simulink model "W2_prob2"  (R2020b)
settings: Solver=VariableStepAuto  StartTime=0.0  StopTime=10.0  RelTol=1e-3
values from neighbouring files (symbols this model uses):
  be = 2.0    [data2_dic.sldd]
  bv = 1.0    [data2_dic.sldd]
  Ie = 1.0    [data2_dic.sldd]
  Iv = 5.0    [data2_dic.sldd]
  R = 1.0    [data2_dic.sldd]
  Uk = 1.0    [data2_dic.sldd]
  Us = 1.5    [data2_dic.sldd]
settings Model: DataDictionary=data2_dic.sldd  Creator=deves  LastModifiedBy=deves
settings SolverCC: ZeroCrossAlgorithm=Adaptive
settings DebuggingCC: IgnoredZcDiagnostic=none

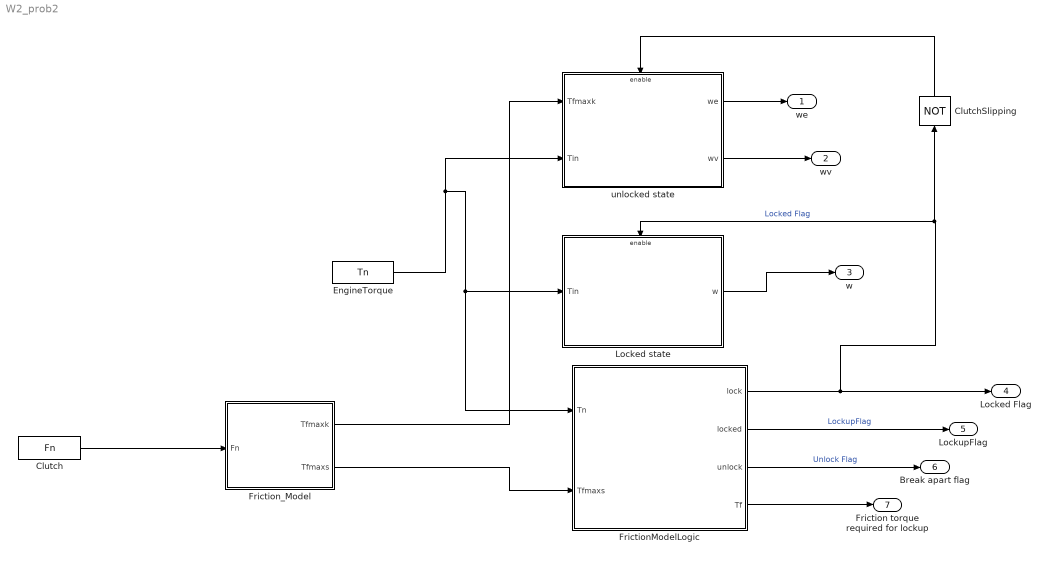
== system W2_prob2 ==
  Clutch : FromWorkspace  VariableName=Fn
  ClutchSlipping : Logic  Operator=NOT  IconShape=distinctive  AllPortsSameDT=off  OutDataTypeStr=boolean
  EngineTorque : FromWorkspace  VariableName=Tn
  FrictionModelLogic : Subsystem
  Friction_Model : Subsystem
  Locked state : Subsystem
  unlocked state : Subsystem
  we : Outport
  wv : Outport  Port=2
  w : Outport  Port=3
  Locked Flag : Outport  Port=4
  LockupFlag : Outport  Port=5
  Break apart flag : Outport  Port=6
  Friction torque required for lockup : Outport  Port=7
  wires:
  Clutch/1 -> Friction_Model/1(Fn)
  EngineTorque/1 -> unlocked state/2(Tin), Locked state/1(Tin), FrictionModelLogic/1(Tn)
  Friction_Model/2(Tfmaxs) -> FrictionModelLogic/2(Tfmaxs)
  unlocked state/1(we) -> we/1
  unlocked state/2(wv) -> wv/1
  Locked state/1(w) -> w/1
  FrictionModelLogic/1(lock) -> ClutchSlipping/1, Locked state/Enable, Locked Flag/1  "Locked Flag"
  FrictionModelLogic/2(locked) -> LockupFlag/1  "LockupFlag"
  FrictionModelLogic/4(Tf) -> Friction torque required for lockup/1
  FrictionModelLogic/3(unlock) -> Break apart flag/1  "Unlock Flag"
  ClutchSlipping/1 -> unlocked state/Enable
  Friction_Model/1(Tfmaxk) -> unlocked state/1(Tfmaxk)

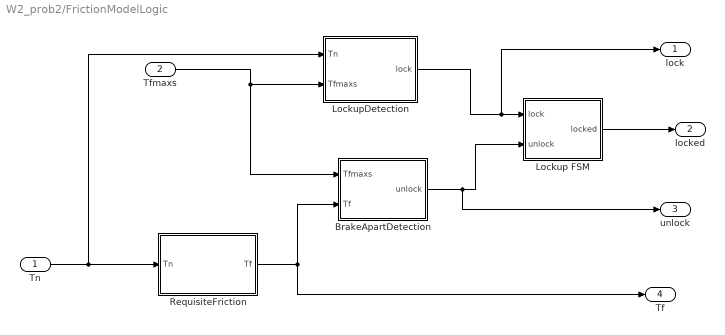
== system W2_prob2/FrictionModelLogic ==
  Tn : Inport
  Tfmaxs : Inport  Port=2
  BrakeApartDetection : Subsystem
  Lockup FSM : Subsystem
  LockupDetection : Subsystem
  RequisiteFriction : Subsystem
  lock : Outport
  locked : Outport  Port=2
  unlock : Outport  Port=3
  Tf : Outport  Port=4
  wires:
  Tn/1 -> LockupDetection/1(Tn), RequisiteFriction/1(Tn)
  LockupDetection/1(lock) -> lock/1, Lockup FSM/1(lock)
  BrakeApartDetection/1(unlock) -> unlock/1, Lockup FSM/2(unlock)
  Tfmaxs/1 -> LockupDetection/2(Tfmaxs), BrakeApartDetection/1(Tfmaxs)
  RequisiteFriction/1(Tf) -> Tf/1, BrakeApartDetection/2(Tf)
  Lockup FSM/1(locked) -> locked/1

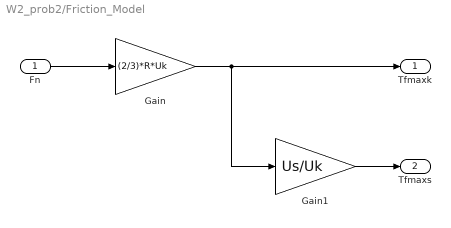
== system W2_prob2/Friction_Model ==
  Fn : Inport
  Gain : Gain  Gain=(2/3)*R*Uk
  Gain1 : Gain  Gain=Us/Uk
  Tfmaxk : Outport
  Tfmaxs : Outport  Port=2
  wires:
  Gain/1 -> Gain1/1, Tfmaxk/1
  Fn/1 -> Gain/1
  Gain1/1 -> Tfmaxs/1

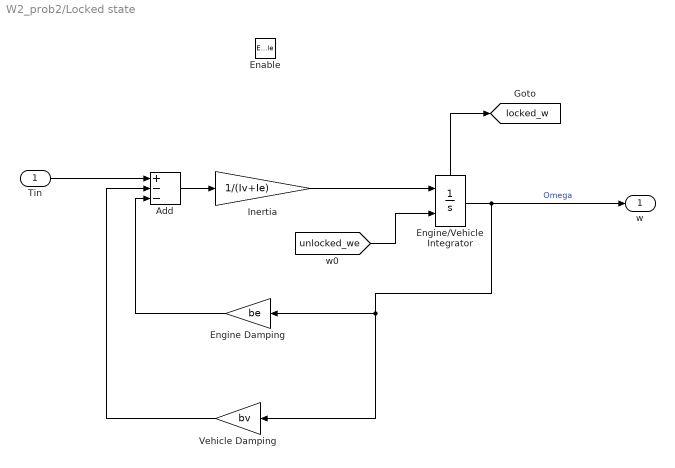
== system W2_prob2/Locked state ==
  Tin : Inport
  Enable : EnablePort  StatesWhenEnabling=reset
  Add : Sum  Inputs=+--
  Engine Damping : Gain  Gain=be  SaturateOnIntegerOverflow=on  OutDataTypeStr=Inherit: Same as input  ParamDataTypeStr=Inherit: Same as input
  Engine/Vehicle Integrator : Integrator  InitialConditionSource=external  ShowStatePort=on
  Inertia : Gain  Gain=1/(Iv+Ie)  SaturateOnIntegerOverflow=on  OutDataTypeStr=Inherit: Same as input  ParamDataTypeStr=Inherit: Same as input
  Vehicle Damping : Gain  Gain=bv  SaturateOnIntegerOverflow=on  OutDataTypeStr=Inherit: Same as input  ParamDataTypeStr=Inherit: Same as input
  w : Outport  InitialOutput=0  VectorParamsAs1DForOutWhenUnconnected=off
  tag scope: locked_w=global
  wires:
  [unlocked_we] -> Engine/Vehicle Integrator/2
  Engine/Vehicle Integrator/1 -> w/1, Engine Damping/1, Vehicle Damping/1  "Omega"
  Inertia/1 -> Engine/Vehicle Integrator/1
  Engine/Vehicle Integrator/State -> [locked_w]
  Add/1 -> Inertia/1
  Tin/1 -> Add/1
  Vehicle Damping/1 -> Add/2
  Engine Damping/1 -> Add/3

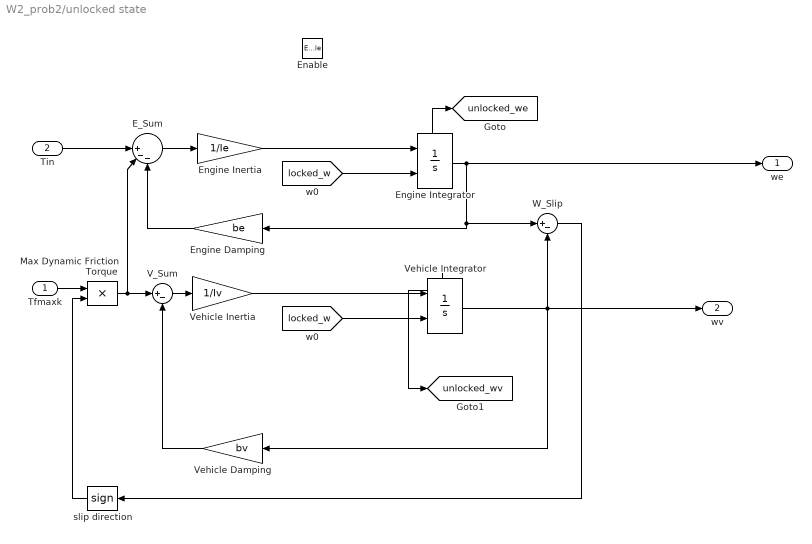
== system W2_prob2/unlocked state ==
  Tfmaxk : Inport
  Tin : Inport  Port=2
  Enable : EnablePort  StatesWhenEnabling=reset
  E_Sum : Sum  Inputs=||+--  InputSameDT=on  SaturateOnIntegerOverflow=on  OutDataTypeStr=Inherit: Same as first input
  Engine Damping : Gain  Gain=be  SaturateOnIntegerOverflow=on  OutDataTypeStr=Inherit: Same as input  ParamDataTypeStr=Inherit: Same as input
  Engine Inertia : Gain  Gain=1/Ie  SaturateOnIntegerOverflow=on  OutDataTypeStr=Inherit: Same as input  ParamDataTypeStr=Inherit: Same as input
  Engine Integrator : Integrator  InitialConditionSource=external  ShowStatePort=on
  Max Dynamic Friction Torque : Product  InputSameDT=on  RndMeth=Zero  SaturateOnIntegerOverflow=on  OutDataTypeStr=Inherit: Same as first input
  V_Sum : Sum  Inputs=|+-  InputSameDT=on  SaturateOnIntegerOverflow=on  OutDataTypeStr=Inherit: Same as first input
  Vehicle Damping : Gain  Gain=bv  SaturateOnIntegerOverflow=on  OutDataTypeStr=Inherit: Same as input  ParamDataTypeStr=Inherit: Same as input
  Vehicle Inertia : Gain  Gain=1/Iv  SaturateOnIntegerOverflow=on  OutDataTypeStr=Inherit: Same as input  ParamDataTypeStr=Inherit: Same as input
  Vehicle Integrator : Integrator  InitialConditionSource=external  ShowStatePort=on
  W_Slip : Sum  Inputs=|+-  InputSameDT=on  SaturateOnIntegerOverflow=on  OutDataTypeStr=Inherit: Same as first input
  slip direction : Signum
  we : Outport  InitialOutput=0  VectorParamsAs1DForOutWhenUnconnected=off
  wv : Outport  Port=2  InitialOutput=0  VectorParamsAs1DForOutWhenUnconnected=off
  tag scope: unlocked_we=global, unlocked_wv=global
  wires:
  W_Slip/1 -> slip direction/1
  [locked_w] -> Vehicle Integrator/2
  Engine Integrator/State -> [unlocked_we]
  Vehicle Damping/1 -> V_Sum/2
  Max Dynamic Friction Torque/1 -> V_Sum/1, E_Sum/2
  Tfmaxk/1 -> Max Dynamic Friction Torque/1
  Vehicle Integrator/1 -> Vehicle Damping/1, wv/1, W_Slip/2
  Vehicle Inertia/1 -> Vehicle Integrator/1
  [locked_w] -> Engine Integrator/2
  E_Sum/1 -> Engine Inertia/1
  Vehicle Integrator/State -> [unlocked_wv]
  Engine Inertia/1 -> Engine Integrator/1
  Engine Damping/1 -> E_Sum/3
  Engine Integrator/1 -> we/1, Engine Damping/1, W_Slip/1
  V_Sum/1 -> Vehicle Inertia/1
  slip direction/1 -> Max Dynamic Friction Torque/2
  Tin/1 -> E_Sum/1

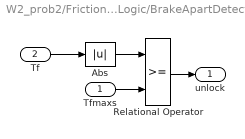
== system W2_prob2/FrictionModelLogic/BrakeApartDetection ==
  Tfmaxs : Inport
  Tf : Inport  Port=2
  Abs : Abs  SaturateOnIntegerOverflow=on
  Relational Operator : RelationalOperator  OutDataTypeStr=boolean  RndMeth=Nearest  InputSameDT=on
  unlock : Outport  InitialOutput=0  VectorParamsAs1DForOutWhenUnconnected=off
  wires:
  Abs/1 -> Relational Operator/1
  Tfmaxs/1 -> Relational Operator/2
  Relational Operator/1 -> unlock/1
  Tf/1 -> Abs/1

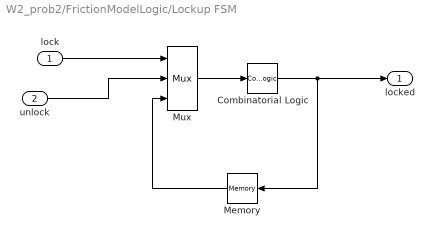
== system W2_prob2/FrictionModelLogic/Lockup FSM ==
  lock : Inport
  unlock : Inport  Port=2
  Combinatorial Logic : CombinatorialLogic  TruthTable=[0;1;0;0;1;1;1;0]
  Memory : Memory
  Mux : Mux  Inputs=3
  locked : Outport  InitialOutput=0  VectorParamsAs1DForOutWhenUnconnected=off
  wires:
  unlock/1 -> Mux/2
  Combinatorial Logic/1 -> locked/1, Memory/1
  Memory/1 -> Mux/3
  Mux/1 -> Combinatorial Logic/1
  lock/1 -> Mux/1

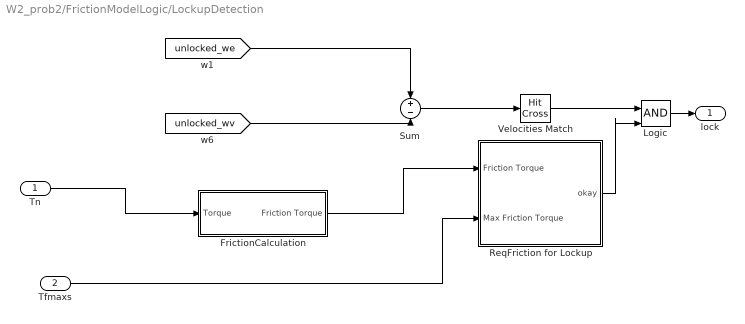
== system W2_prob2/FrictionModelLogic/LockupDetection ==
  Tn : Inport
  Tfmaxs : Inport  Port=2
  FrictionCalculation : Subsystem
  Logic : Logic  IconShape=distinctive  OutDataTypeStr=boolean
  ReqFriction for Lockup : Subsystem
  Sum : Sum  Inputs=+-  InputSameDT=on  SaturateOnIntegerOverflow=on  OutDataTypeStr=Inherit: Same as first input
  Velocities Match : HitCross
  lock : Outport  InitialOutput=0  VectorParamsAs1DForOutWhenUnconnected=off
  wires:
  [unlocked_wv] -> Sum/2
  Logic/1 -> lock/1
  Sum/1 -> Velocities Match/1
  Velocities Match/1 -> Logic/1
  [unlocked_we] -> Sum/1
  ReqFriction for Lockup/1(okay) -> Logic/2
  FrictionCalculation/1(Friction Torque) -> ReqFriction for Lockup/1(Friction Torque)
  Tfmaxs/1 -> ReqFriction for Lockup/2(Max Friction Torque)
  Tn/1 -> FrictionCalculation/1(Torque)

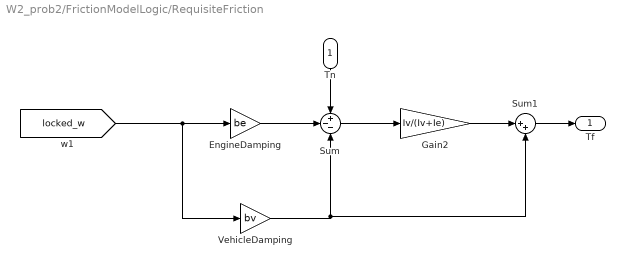
== system W2_prob2/FrictionModelLogic/RequisiteFriction ==
  Tn : Inport
  EngineDamping : Gain  Gain=be
  Gain2 : Gain  Gain=Iv/(Iv+Ie)
  Sum : Sum  Inputs=+--
  Sum1 : Sum  Inputs=|++
  VehicleDamping : Gain  Gain=bv
  Tf : Outport
  wires:
  VehicleDamping/1 -> Sum1/2, Sum/3
  EngineDamping/1 -> Sum/2
  [locked_w] -> VehicleDamping/1, EngineDamping/1
  Sum/1 -> Gain2/1
  Tn/1 -> Sum/1
  Gain2/1 -> Sum1/1
  Sum1/1 -> Tf/1

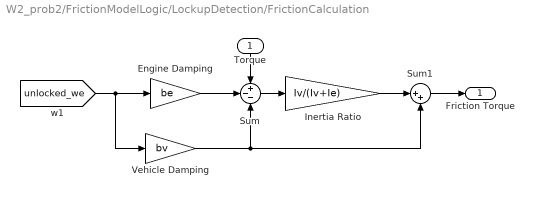
== system W2_prob2/FrictionModelLogic/LockupDetection/FrictionCalculation ==
  Torque : Inport
  Engine Damping : Gain  Gain=be  SaturateOnIntegerOverflow=on  OutDataTypeStr=Inherit: Same as input  ParamDataTypeStr=Inherit: Same as input
  Inertia Ratio : Gain  Gain=Iv/(Iv+Ie)  SaturateOnIntegerOverflow=on  OutDataTypeStr=Inherit: Same as input  ParamDataTypeStr=Inherit: Same as input
  Sum : Sum  Inputs=+--  InputSameDT=on  SaturateOnIntegerOverflow=on  OutDataTypeStr=Inherit: Same as first input
  Sum1 : Sum  Inputs=|++  InputSameDT=on  SaturateOnIntegerOverflow=on  OutDataTypeStr=Inherit: Same as first input
  Vehicle Damping : Gain  Gain=bv  SaturateOnIntegerOverflow=on  OutDataTypeStr=Inherit: Same as input  ParamDataTypeStr=Inherit: Same as input
  Friction Torque : Outport  InitialOutput=0  VectorParamsAs1DForOutWhenUnconnected=off
  wires:
  Sum1/1 -> Friction Torque/1
  Torque/1 -> Sum/1
  Inertia Ratio/1 -> Sum1/1
  Vehicle Damping/1 -> Sum1/2, Sum/3
  [unlocked_we] -> Engine Damping/1, Vehicle Damping/1
  Engine Damping/1 -> Sum/2
  Sum/1 -> Inertia Ratio/1

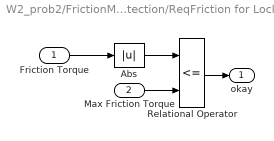
== system W2_prob2/FrictionModelLogic/LockupDetection/ReqFriction for Lockup ==
  Friction Torque : Inport
  Max Friction Torque : Inport  Port=2
  Abs : Abs  SaturateOnIntegerOverflow=on
  Relational Operator : RelationalOperator  Operator=<=  OutDataTypeStr=boolean  RndMeth=Nearest  InputSameDT=on
  okay : Outport  InitialOutput=0  VectorParamsAs1DForOutWhenUnconnected=off
  wires:
  Friction Torque/1 -> Abs/1
  Abs/1 -> Relational Operator/1
  Relational Operator/1 -> okay/1
  Max Friction Torque/1 -> Relational Operator/2
